simulink model "E_poa"  (R2025b)
settings: Solver=VariableStepAuto  StartTime=0.0  StopTime=1440  RelTol=1e-3
undefined symbols (not defined in the file or in its folder): panel
settings Model: Creator=krist  LastModifiedBy=krist

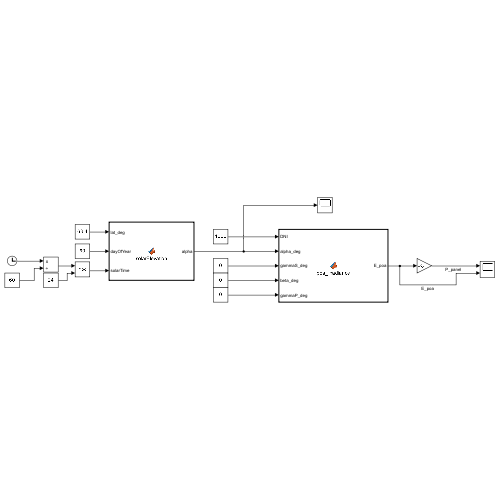
[thumbnail: Simulink's stored preview of the top-level diagram]
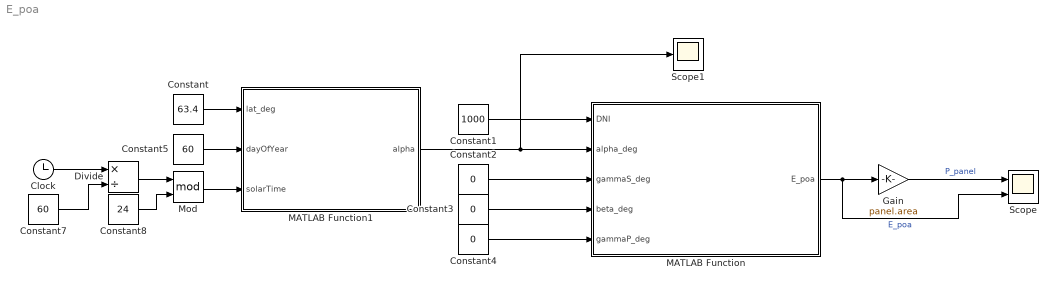
== system E_poa ==
  Clock : Clock
  Constant : Constant  Value=63.4
  Constant1 : Constant  Value=1000
  Constant2 : Constant  Value=0
  Constant3 : Constant  Value=0
  Constant4 : Constant  Value=0
  Constant5 : Constant  Value=60
  Constant7 : Constant  Value=60
  Constant8 : Constant  Value=24
  Divide : Product  Inputs=*/
  Gain : Gain  Gain=panel.area
  MATLAB Function : MATLAB Function  TreatAsAtomicUnit=on
  MATLAB Function1 : MATLAB Function  TreatAsAtomicUnit=on
  Mod : Math  Operator=mod
  Scope : Scope  NumInputPorts=2
      settings: ActiveDisplayYMinimum=-392.6209561564151  ActiveDisplayYMaximum=3533.5886054077368  YLabel=Power W
  Scope1 : Scope
      settings: ActiveDisplayYMinimum=-55.199965386315277  ActiveDisplayYMaximum=56.26208813539268
  wires:
  MATLAB Function/1(E_poa) -> Scope/2, Gain/1  "E_poa"
  MATLAB Function1/1(alpha) -> Scope1/1, MATLAB Function/2(alpha_deg)
  Constant1/1 -> MATLAB Function/1(DNI)
  Constant2/1 -> MATLAB Function/3(gammaS_deg)
  Constant3/1 -> MATLAB Function/4(beta_deg)
  Constant4/1 -> MATLAB Function/5(gammaP_deg)
  Gain/1 -> Scope/1  "P_panel"
  Constant/1 -> MATLAB Function1/1(lat_deg)
  Constant5/1 -> MATLAB Function1/2(dayOfYear)
  Mod/1 -> MATLAB Function1/3(solarTime)
  Clock/1 -> Divide/1
  Constant7/1 -> Divide/2
  Divide/1 -> Mod/1
  Constant8/1 -> Mod/2

== matlab function E_poa/MATLAB Function1 ==
  data: lat_deg input; alpha output; dayOfYear input; solarTime input
function alpha = solarElevation(lat_deg, dayOfYear, solarTime)
% SOLARELEVATION  Solar elevation angle (degrees)
%
% lat_deg    : latitude [deg] (e.g. Trondheim = 63.4)
% dayOfYear  : day number (March 1 = 60, March 21 ≈ 80)
% solarTime  : solar time [hours] (solar noon = 12)

phi = deg2rad(lat_deg);

% Solar declination
delta = deg2rad(23.45 * sind(360*(284 + dayOfYear)/365));

% Hour angle
h = deg2rad(15*(solarTime - 12));

% Solar elevation angle
alpha = asind( ...
    sin(phi).*sin(delta) + ...
    cos(phi).*cos(delta).*cos(h) ...
);
end

== matlab function E_poa/MATLAB Function ==
  data: DNI input; E_poa output; alpha_deg input; gammaS_deg input; beta_deg input; gammaP_deg input
function E_poa = poa_irradiance(DNI, alpha_deg, gammaS_deg, beta_deg, gammaP_deg)
% Plane-of-array irradiance from direct normal irradiance and angles.
% Inputs in degrees, DNI in W/m^2. Output E_poa in W/m^2.

alpha = deg2rad(alpha_deg);
beta  = deg2rad(beta_deg);
dgam  = deg2rad(gammaS_deg - gammaP_deg);

theta_z = pi/2 - alpha;

cosAOI = cos(theta_z).*cos(beta) + sin(theta_z).*sin(beta).*cos(dgam);
cosAOI = max(cosAOI, 0);   % if sun behind panel

E_poa = DNI .* cosAOI;
end
